simulink model "DistanceTest"  (R2018b)
settings: Solver=ode3  StartTime=0.0  StopTime=10  RelTol=1e-3  EnableMultiTasking=on
undefined symbols (not defined in the file): Stateflow
libraries: legoev3lib x2, DistanceSensor x1
settings Model: FPTRunName=Active  ExtModeTrigDuration=2  Creator=nico  LastModifiedBy=nico
settings SolverCC: PositivePriorityOrder=on
settings DataIOCC: LimitDataPoints=on  SaveFormat=Array
settings OptimizationCC: ExpressionDepthLimit=2147483647  LifeSpan=Inf  MaxStackSize=64
settings DebuggingCC: UnderspecifiedInitializationDetection=Classic  MergeDetectMultiDrivingBlocksExec=none  FcnCallInpInsideContextMsg=warning  AllowSymbolicDim=off  StateNameClashWarn=warning  SFUnexpectedBacktrackingDiag=warning  SFNoUnconditionalDefaultTransitionDiag=warning  SFExecutionAtInitializationDiag=none
settings HardwareCC: ProdBitPerPointer=32  ProdBitPerSizeT=32  ProdBitPerPtrDiffT=32  ProdLargestAtomicInteger=Long  ProdWordSize=32  ProdHWDeviceType=ARM Compatible->ARM 9  UseEmbeddedCoderFeatures=off  UseSimulinkCoderFeatures=off
settings ModelReferenceCC: PropagateSignalLabelsOutOfModel=off
settings SFSimCC: SimUseLocalCustomCode=off
settings RTWCC: SystemTargetFile=ert.tlc  HardwareBoard=LEGO MINDSTORMS EV3  TemplateMakefile=ert_default_tmf  GenerateReport=on  RTWVerbose=off  RTWUseLocalCustomCode=off  Toolchain=Sourcery G++ Lite v2009q3  BuildConfiguration=Faster Runs  LaunchReport=on
settings CodeAppCC: ForceParamTrailComments=on  OperatorAnnotations=on  StateflowObjectComments=on  MATLABSourceComments=on
settings ERTTargetCC: MultiwordLength=2048  ERTCustomFileBanners=off  SupportContinuousTime=on  SupportNonInlinedSFcns=on  RemoveResetFunc=off  SupportVariableSizeSignals=on  ModelStepFunctionPrototypeControlCompliant=off
settings ConfigComp: CovMetricSettings=dw  CovHtmlReporting=on  CovSaveCumulativeToWorkspaceVar=on  CovSaveSingleToWorkspaceVar=on  CovExternalEMLEnable=off  CovSFcnEnable=off

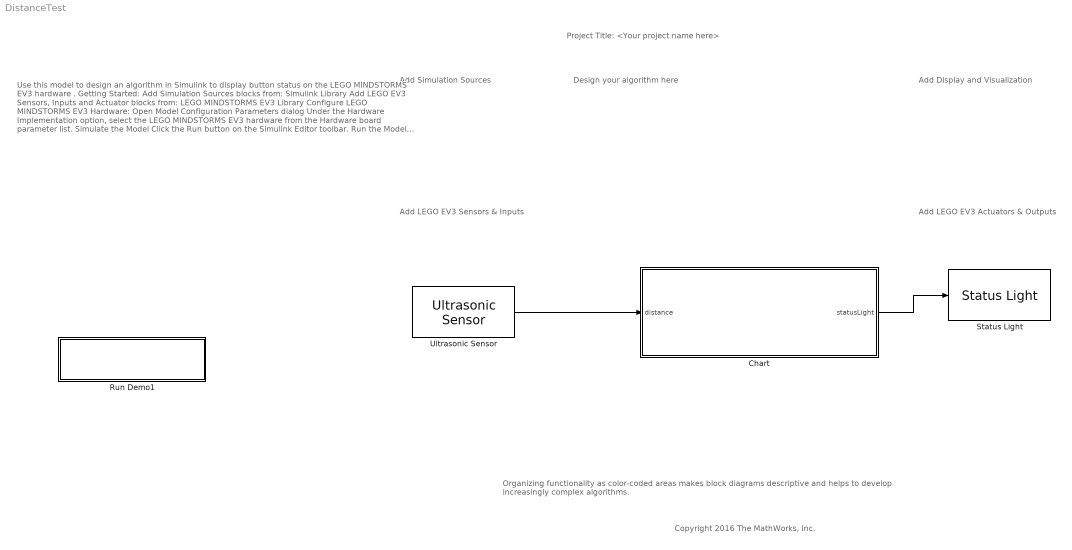
== system DistanceTest ==
  note: Project Title: <Your project name here>
  note: Copyright 2016 The MathWorks, Inc.
  note: Add LEGO EV3 Sensors & Inputs
  note: Add LEGO EV3 Actuators & Outputs
  note: Add Display and Visualization
  note: Design your algorithm here
  note: Add Simulation Sources
  note: Use this model to design an algorithm in Simulink to display button status on the LEGO MINDSTORMS EV3 hardware .
      |
      | Getting Started:
      |
      | Add Simulation Sources blocks from:
      | Simulink Library
      | Add LEGO EV3 Sensors, Inputs and Actuator blocks from:
      | LEGO MINDSTORMS EV3 Library
      |
      | Configure LEGO MINDSTORMS EV3 Hardware:
      |
      | Open Model Configuration Parameters dialog
      | Under the Hardware Implementation option, select the LEGO MINDSTORMS EV3 hardware from the Hardware board parameter list.
      |
      | Simulate the Model
      |
      | Click the Run button on the Simulink Editor toolbar.
      |
      | Run the Model on LEGO MINDSTORMS EV3 Hardware
      |
      | Click the Deploy to Hardware button on the Simulink Editor toolbar.
      |
      | Other Things to Try:
      |
      | Create and run a model that detects the obstacle and stops the LEGO EV3 robot. HINT: Use Ultrasonic Sensor and Motor blocks.
  note: Organizing functionality as color-coded areas makes block diagrams descriptive and helps to develop increasingly complex algorithms.
  Chart : Stateflow chart  TreatAsAtomicUnit=on
  Run Demo1 : Subsystem  Description=Controls host-side RTDX processing.
      mask Display: pic=imread('ev3DeploytoHardware.png');image(pic);
  Status Light : legoev3lib/Status Light
      settings: SourceProductName=Simulink Support Package for LEGO MINDSTORMS EV3 Hardware  SourceProductBaseCode=LEGOEV3
  Ultrasonic Sensor : legoev3lib/Ultrasonic Sensor  PortNumber=4  sampleTime=0.1
      settings: SourceProductName=Simulink Support Package for LEGO MINDSTORMS EV3 Hardware  SourceProductBaseCode=LEGOEV3
  wires:
  Chart/1(statusLight) -> Status Light/1
  Ultrasonic Sensor/1 -> Chart/1(distance)

== system DistanceTest/Run Demo1 ==

== stateflow chart DistanceTest/Chart ==
  state Distance_Sensor [parallel]
    settings: executionOrder=1
  state StatusBLaBla [parallel]
    entry: statusLight = 0
    settings: executionOrder=2
    state AtEase
    state ToClose
      entry: statusLight = 2
    state FoundBeast
      entry: statusLight = 3
    state Approaching
      entry: statusLight = 1
    (default) -> AtEase
    AtEase -> ToClose [order 1] : [TOO_CLOSE_TO_BEAST]
    ToClose -> AtEase
    AtEase -> FoundBeast [order 2] : [FOUND_BEAST]
    AtEase -> Approaching [order 3] : [APPROACHING_BEAST]
    Approaching -> AtEase
    FoundBeast -> AtEase
  (default) -> StatusBLaBla
  data: FOUND_BEAST function_output; APPROACHING_BEAST function_output; TOO_CLOSE_TO_BEAST function_output; statusLight output uint32 size=1; distance input uint8 size=1; FOUND_BEAST local boolean size=1; TOO_CLOSE_TO_BEAST local boolean size=1; APPROACHING_BEAST local boolean size=1
